simulink model "mainModel"  (R2022a)
settings: Solver=VariableStepAuto  StartTime=0.0  StopTime=10.0  RelTol=1e-3
model workspace (MAT data in the model file):
  Jr = Simulink.Parameter
  Jr.Value = 6.5e-07
  Jr.DataType = 'double'
  Jr.Complexity = 'real'
  Jr.Dimensions = [1 1]
  Kemf = Simulink.Parameter
  Kemf.Value = 0.00255
  Kemf.DataType = 'double'
  Kemf.Complexity = 'real'
  Kemf.Dimensions = [1 1]
  Kt = Simulink.Parameter
  Kt.Value = 0.00255
  Kt.DataType = 'double'
  Kt.Complexity = 'real'
  Kt.Dimensions = [1 1]
  L = Simulink.Parameter
  L.Value = 0.000117
  L.DataType = 'double'
  L.Complexity = 'real'
  L.Dimensions = [1 1]
  R = Simulink.Parameter
  R.Value = 0.17
  R.DataType = 'double'
  R.Complexity = 'real'
  R.Dimensions = [1 1]
  b_m = Simulink.Parameter
  b_m.Value = 2.415e-06
  b_m.DataType = 'double'
  b_m.Complexity = 'real'
  b_m.Dimensions = [1 1]
  g = Simulink.Parameter
  g.Value = -9.81
  g.DataType = 'double'
  g.Complexity = 'real'
  g.Dimensions = [1 1]
  kt = 2.64e-08
  m = Simulink.Parameter
  m.Value = 0.05656
  m.DataType = 'double'
  m.Complexity = 'real'
  m.Dimensions = [1 1]
settings Model: Creator=danfo  LastModifiedBy=danfo

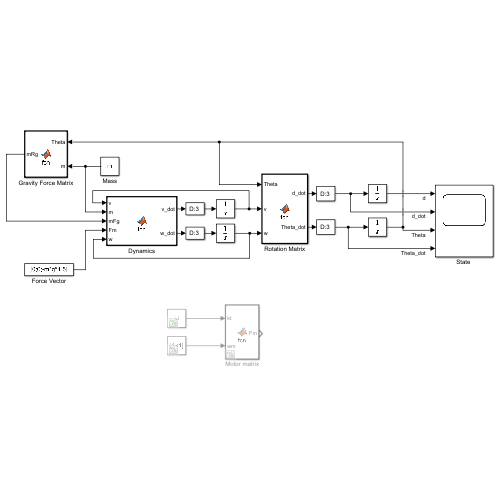
[thumbnail: Simulink's stored preview of the top-level diagram]
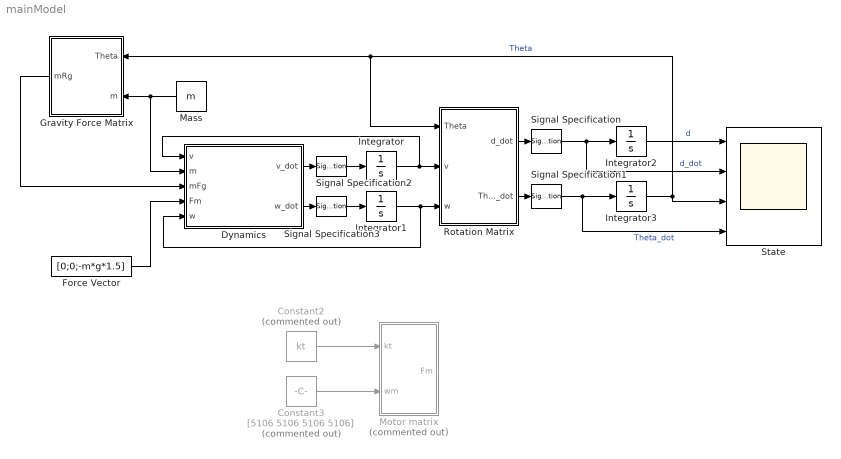
== system mainModel ==
  Constant2 : Constant  Commented=on  Value=kt
  Constant3 : Constant  Commented=on  Value=[5106 5106 5106 5106]
  Dynamics : MATLAB Function  TreatAsAtomicUnit=on
  Force Vector : Constant  Value=[0;0;-m*g*1.5]
  Gravity Force Matrix : MATLAB Function  TreatAsAtomicUnit=on
  Integrator{,1..3} (4 alike) : Integrator
  Mass : Constant  Value=m
  Motor matrix : MATLAB Function  Commented=on  TreatAsAtomicUnit=on
  Rotation Matrix : MATLAB Function  TreatAsAtomicUnit=on
  Signal Specification{,1..3} (4 alike) : SignalSpecification  Dimensions=3
  "State " : Scope  NumInputPorts=4
  wires:
  Constant2/1 -> Motor matrix/1(kt)
  Constant3/1 -> Motor matrix/2(wm)
  Mass/1 -> Dynamics/2(m), Gravity Force Matrix/2(m)
  Integrator1/1 -> Dynamics/5(w), Rotation Matrix/3(w)
  Rotation Matrix/1(d_dot) -> Signal Specification/1
  Rotation Matrix/2(Theta_dot) -> Signal Specification1/1
  Integrator3/1 -> Rotation Matrix/1(Theta), Gravity Force Matrix/1(Theta), "State "/3  "Theta"
  Integrator/1 -> Dynamics/1(v), Rotation Matrix/2(v)
  Integrator2/1 -> "State "/1  "d"
  Signal Specification/1 -> "State "/2, Integrator2/1  "d_dot"
  Signal Specification1/1 -> "State "/4, Integrator3/1  "Theta_dot"
  Signal Specification2/1 -> Integrator/1
  Dynamics/1(v_dot) -> Signal Specification2/1
  Dynamics/2(w_dot) -> Signal Specification3/1
  Signal Specification3/1 -> Integrator1/1
  Force Vector/1 -> Dynamics/4(Fm)
  Gravity Force Matrix/1(mRg) -> Dynamics/3(mFg)

== matlab function mainModel/Dynamics ==
  data: v input; m input; mFg input; Fm input; v_dot output; w input; w_dot output
function [v_dot, w_dot] = fcn(v, m, mFg, Fm, w)

v_dot = ((Fm + m.*mFg)./m)-(cross(v,w));

w_dot = [0,0,0];

== matlab function mainModel/Gravity Force Matrix ==
  data: Theta input; mRg output; m input
function mRg  = fcn (Theta, m)

phi = Theta(1);
theta = Theta(2);
g = -9.81;

mRg = [-m*g*sind(theta); m*g*cosd(theta)*sind(phi); m*g*cosd(theta)*cosd(phi)];

== matlab function mainModel/Motor matrix ==
  data: kt input; Fm output; wm input
function Fm = fcn(kt, wm)

F_sum = -(kt.*wm(1) + kt.*wm(2) +kt.*wm(3) +kt.*wm(4));
Fm = [0;0;F_sum];

== matlab function mainModel/Rotation Matrix ==
  data: Theta input; d_dot output; Theta_dot output; v input; w input
function [d_dot,Theta_dot] = fcn(Theta, v, w)

phi = Theta(1);
theta = Theta(2);
psi = Theta(3);

% Linear velocity rotation matrix: 3x3 --> 9 elements
R_1 = [cosd(psi)*cosd(theta), -cosd(phi)*sind(psi)+cosd(psi)*sind(phi)*sind(theta), sind(phi)*sind(psi)+cosd(phi)*cosd(psi)*(sind(theta));
cosd(theta)*sind(psi), cosd(phi)*cosd(psi)+sind(psi)*sind(theta)*sind(phi), -cosd(psi)*sind(phi)+sind(psi)*sind(theta)*cosd(phi);
-sind(theta), cosd(theta)*sind(phi), cosd(theta)*cosd(phi)];

% Angular velocity rotation matrix
R_2 = [1, sind(phi)*tand(theta), cosd(phi)*tand(theta);
0, cosd(phi), -sind(phi);
0, sind(phi)/cosd(theta), cosd(phi)/cosd(theta)];

d_dot = R_1*v;
Theta_dot= R_2*w;
